simulink model "AdaptiveThreshold"  (R2020a)
settings: Solver=VariableStepAuto  StartTime=0  StopTime=10  RelTol=1e-3
values from neighbouring files (symbols this model uses):
  feature_buffer = fs    (= 30000)    [run_AdaptiveThreshold.m]    (also in run_AdaptiveThresholdLocalMaxima.m; run_LocalMaxima_AdaptiveThreshold.m; run_Sample_AdaptiveThreshold.m)
  feature_gain = [1, 3, 5, 7]    [run_AdaptiveThreshold.m]    (also in run_AdaptiveThresholdLocalMaxima.m = [1 3 5 7]; run_LocalMaxima_AdaptiveThreshold.m = [1:0.25:7]; run_Sample_AdaptiveThreshold.m = [7]; run_SigmaDelta_AdaptiveThreshold.m = [5])
  fs = 30000    [run_AdaptiveThreshold.m]    (also in run_AdaptiveThresholdLocalMaxima.m; run_HardThreshold.m; run_HardThresholdLocalMaxima.m; run_LocalMaxima_AdaptiveThreshold.m)
  refractory = 10^-3    (= 0.001)    [run_AdaptiveThreshold.m]    (also in run_AdaptiveThresholdLocalMaxima.m; run_HardThreshold.m; run_HardThresholdLocalMaxima.m; run_LocalMaxima_AdaptiveThreshold.m)
libraries: dspfdesign x2, dspswit3 x1, dspstat3 x1, simulink x1, hdlsllib x1
settings Model: Creator=sbuccelli  LastModifiedBy=diflo

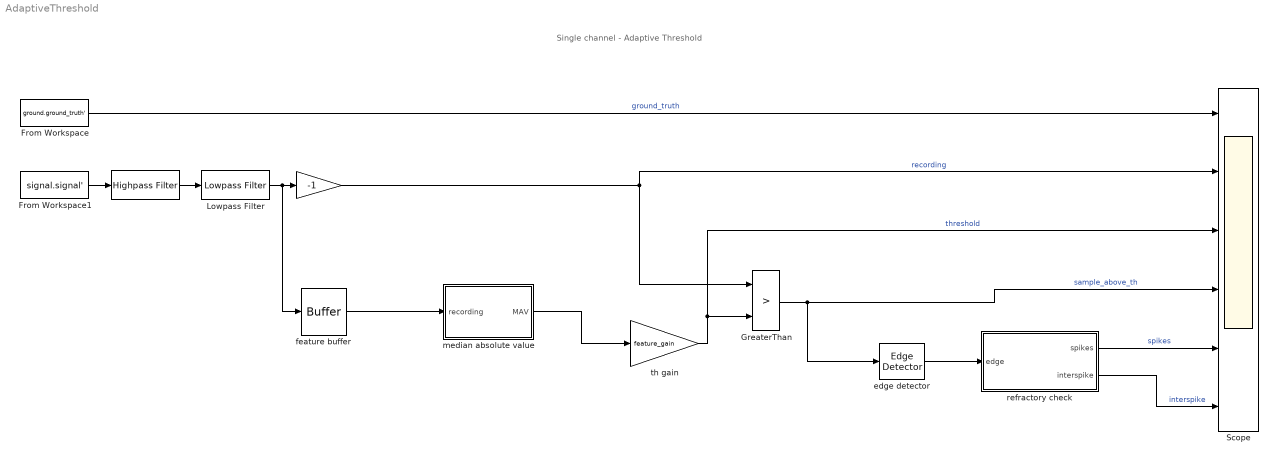
== system AdaptiveThreshold ==
  note: Single channel - Adaptive Threshold
  " " : Gain  Gain=-1
  "   " : dspfdesign/Highpass Filter  FilterType=IIR  DesignForMinimumOrder=on  FilterOrder=50  StopbandFrequency=1  PassbandFrequency=300  StopbandAttenuation=80  PassbandRipple=0.1  InheritSampleRate=off  SampleRate=fs  SimulateUsing=Interpreted execution  roundingMode=Floor  coeffsDataTypeStr=fixdt(1,16)
  From Workspace : FromWorkspace  VariableName=ground.ground_truth'  SampleTime=1/fs
  From Workspace1 : FromWorkspace  VariableName=signal.signal'  SampleTime=1/fs
  GreaterThan : RelationalOperator  Operator=>  OutDataTypeStr=boolean  RndMeth=Simplest
  Lowpass Filter : dspfdesign/Lowpass Filter  FilterType=IIR  DesignForMinimumOrder=on  FilterOrder=3  PassbandFrequency=3500  StopbandFrequency=8500  PassbandRipple=0.1  StopbandAttenuation=80  InheritSampleRate=off  SampleRate=fs  SimulateUsing=Interpreted execution  roundingMode=Floor  coeffsDataTypeStr=fixdt(1,16)
  Scope : Scope  NumInputPorts=6
  edge detector : dspswit3/Edge Detector  InputProcessing=Columns as channels (frame based)
      settings: SourceProductBaseCode=DS
  feature buffer : Buffer  N=feature_buffer  OutputFrames=off
  median absolute value : Subsystem
  refractory check : Subsystem
  th gain : Gain  Gain=feature_gain
  wires:
  edge detector/1 -> refractory check/1(" edge ")
  refractory check/2(interspike) -> Scope/6  "interspike"
  GreaterThan/1 -> Scope/4, edge detector/1  "sample_above_th"
  th gain/1 -> GreaterThan/2, Scope/3  "threshold"
  refractory check/1(spikes) -> Scope/5  "spikes"
  Lowpass Filter/1 -> feature buffer/1, " "/1
  " "/1 -> GreaterThan/1, Scope/2  "recording"
  feature buffer/1 -> median absolute value/1(recording)
  median absolute value/1(MAV) -> th gain/1
  From Workspace1/1 -> "   "/1
  From Workspace/1 -> Scope/1  "ground_truth"
  "   "/1 -> Lowpass Filter/1

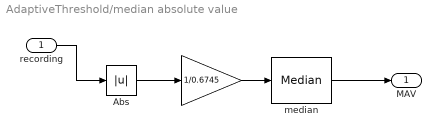
== system AdaptiveThreshold/median absolute value ==
  recording : Inport
  "  " : Gain  Gain=1/0.6745
  Abs : Abs
  median : dspstat3/Median  sortAlg=Quick sort  directionMode=Each column  dimension=1  roundingMode=Floor  overflowMode=off  accumDataTypeStr=Inherit: Same as product output  accumLastDataTypeStr=Inherit: Same as product output  outputDataTypeStr=Inherit: Same as accumulator  outputMin=[]  outputMax=[]  outputLastDataTypeStr=Inherit: Same as accumulator
      settings: SourceProductBaseCode=DS  allowOverrides=off
  MAV : Outport
  wires:
  Abs/1 -> "  "/1
  "  "/1 -> median/1
  recording/1 -> Abs/1
  median/1 -> MAV/1

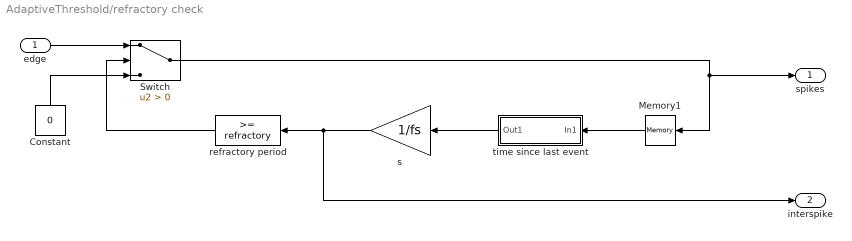
== system AdaptiveThreshold/refractory check ==
  " edge " : Inport
  Constant : Constant  Value=0
  Memory1 : Memory  InheritSampleTime=on
  Switch : Switch  Criteria=u2 > Threshold
  refractory period : simulink/Logic and Bit Operations/Compare To Constant  relop=>=  const=refractory  OutDataTypeStr=boolean
  s : Gain  Gain=1/fs  ParamDataTypeStr=double
  time since last event : Subsystem
  spikes : Outport
  interspike : Outport  Port=2
  wires:
  " edge "/1 -> Switch/1
  Memory1/1 -> time since last event/1(In1)
  time since last event/1(Out1) -> s/1
  Constant/1 -> Switch/3
  s/1 -> refractory period/1, interspike/1
  Switch/1 -> spikes/1, Memory1/1
  refractory period/1 -> Switch/2

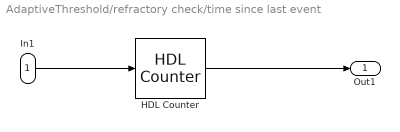
== system AdaptiveThreshold/refractory check/time since last event ==
  In1 : Inport
  HDL Counter : hdlsllib/Sources/HDL Counter  CountType=Free running  CountInit=1  CountStep=1  CountMax=25  CountFromType=Initial value  CountFrom=1  CountResetPort=on  CountLoadPort=off  CountEnbPort=off  CountDirPort=off  CountDataType=Unsigned  CountWordLen=32  CountFracLen=0  CountSampTime=1
  Out1 : Outport
  wires:
  In1/1 -> HDL Counter/1
  HDL Counter/1 -> Out1/1
